simulink model "Part5_6"  (R2022b)
settings: Solver=VariableStepAuto  StartTime=0.0  StopTime=10.0  RelTol=1e-3
settings Model: Creator=NourAldin  LastModifiedBy=NourAldin

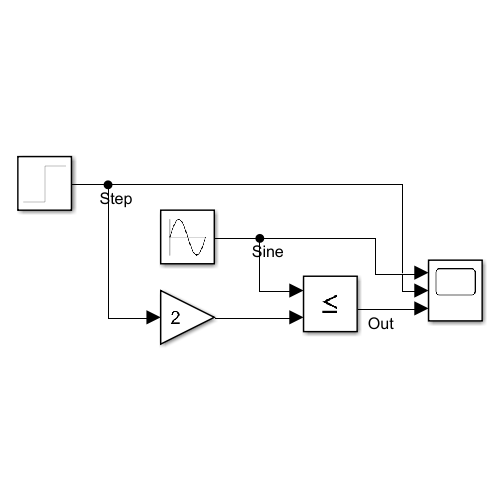
[thumbnail: Simulink's stored preview of the top-level diagram]
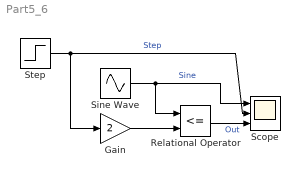
== system Part5_6 ==
  Gain : Gain  Gain=2
  Relational Operator : RelationalOperator  Operator=<=  OutDataTypeStr=boolean  RndMeth=Simplest  InputSameDT=off
  Scope : Scope  NumInputPorts=3
  Sine Wave : Sin  Frequency=1/2*pi  SampleTime=0
  Step : Step  Time=2  SampleTime=0
  wires:
  Step/1 -> Scope/2, Gain/1  "Step"
  Sine Wave/1 -> Scope/1, Relational Operator/1  "Sine"
  Gain/1 -> Relational Operator/2
  Relational Operator/1 -> Scope/3  "Out"
